simulink model "controlPID2"  (R2019a)
settings: Solver=VariableStepAuto  StartTime=0.0  StopTime=15  RelTol=1e-3
values from neighbouring files (symbols this model uses):
  A = [0, 0, 1, 0 ... (first row only)    [Base_proyecto.m]    (also in lqr_proyecto.m)
  B = [0 ... (first row only)    [Base_proyecto.m]    (also in lqr_proyecto.m)
  x0 = [0;5*pi/180; 0; 0]    [Base_proyecto.m]    (also in lqr_proyecto.m)
libraries: simulink x1
settings Model: Creator=WALTER  LastModifiedBy=WALTER

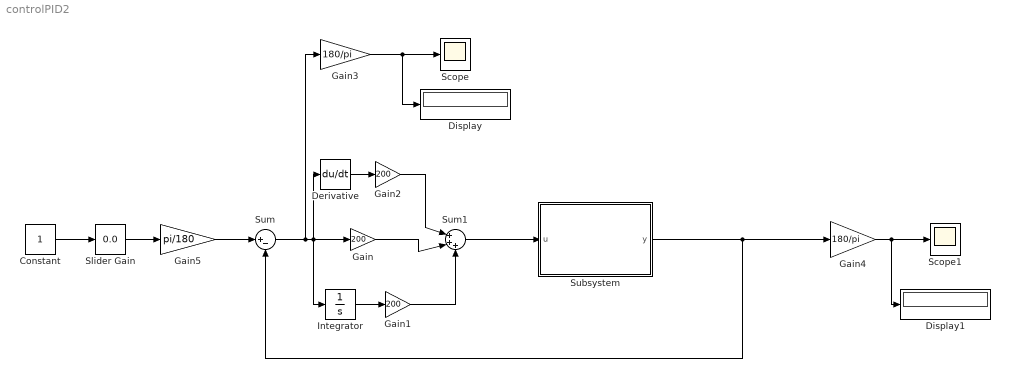
== system controlPID2 ==
  Constant : Constant
  Derivative : Derivative
  Display : Display
  Display1 : Display
  Gain : Gain  Gain=200
  Gain1 : Gain  Gain=200
  Gain2 : Gain  Gain=200
  Gain3 : Gain  Gain=180/pi
  Gain4 : Gain  Gain=180/pi
  Gain5 : Gain  Gain=pi/180
  Integrator : Integrator
  Scope : Scope
  Scope1 : Scope
  Slider Gain : simulink/Math Operations/Slider Gain  gain=0.0  low=-20  high=20
  Subsystem : Subsystem
  Sum : Sum  Inputs=|+-
  Sum1 : Sum  Inputs=|+++
  wires:
  Sum/1 -> Gain3/1, Integrator/1, Gain/1, Derivative/1
  Derivative/1 -> Gain2/1
  Gain2/1 -> Sum1/1
  Gain/1 -> Sum1/2
  Gain1/1 -> Sum1/3
  Integrator/1 -> Gain1/1
  Slider Gain/1 -> Gain5/1
  Constant/1 -> Slider Gain/1
  Gain3/1 -> Display/1, Scope/1
  Gain4/1 -> Display1/1, Scope1/1
  Gain5/1 -> Sum/1
  Sum1/1 -> Subsystem/1(u)
  Subsystem/1(y) -> Sum/2, Gain4/1

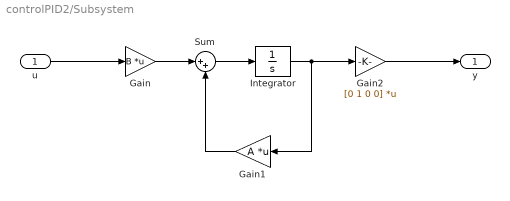
== system controlPID2/Subsystem ==
  u : Inport
  Gain : Gain  Gain=B  Multiplication=Matrix(K*u)
  Gain1 : Gain  Gain=A  Multiplication=Matrix(K*u) (u vector)
  Gain2 : Gain  Gain=[0 1 0 0]  Multiplication=Matrix(K*u) (u vector)
  Integrator : Integrator  InitialCondition=x0
  Sum : Sum  Inputs=|++
  y : Outport
  wires:
  Gain1/1 -> Sum/2
  Gain/1 -> Sum/1
  Integrator/1 -> Gain1/1, Gain2/1
  Gain2/1 -> y/1
  Sum/1 -> Integrator/1
  u/1 -> Gain/1
